simulink model "lab1simulink"  (R2021a)
settings: Solver=VariableStepAuto  StartTime=0.0  StopTime=80  RelTol=1e-3
undefined symbols (not defined in the file): c, d, g, J, L, m
libraries: fuzblock x2, simulink_extras x2
settings Model: Creator=ejbejaranos  LastModifiedBy=ejbejaranos

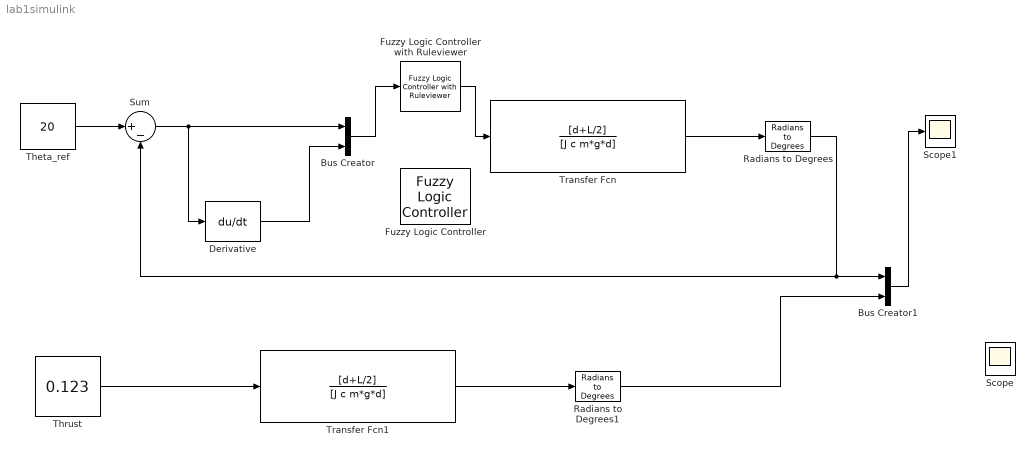
== system lab1simulink ==
  Bus Creator : BusCreator  Inputs=2
  Bus Creator1 : BusCreator  Inputs=2
  Derivative : Derivative
  Fuzzy Logic Controller : fuzblock/Fuzzy Logic  Controller  FIS=Fuzzy  OutputSampleNumber=101  DataType=double  FuzzifiedInputs=off  RuleFiringStrengths=off  RuleOutputs=off  AggregatedOutputs=off  SimulateUsing=Interpreted execution  OutOfRangeInputValueMessage=warning  NoRuleFiredMessage=warning  EmptyOutputFuzzySetMessage=warning
  Fuzzy Logic Controller with Ruleviewer : fuzblock/Fuzzy Logic  Controller  with Ruleviewer  fismatrix=Fuzzy  Ts=2
  Radians to Degrees : simulink_extras/Transformations/Radians to Degrees
  Radians to Degrees1 : simulink_extras/Transformations/Radians to Degrees
  Scope : Scope  NumInputPorts=2
  Scope1 : Scope
  Sum : Sum  Inputs=|+-
  Theta_ref : Constant  Value=20
  Thrust : Constant  Value=0.123
  Transfer Fcn : TransferFcn  Numerator=[d+L/2]  Denominator=[J c m*g*d]
  Transfer Fcn1 : TransferFcn  Numerator=[d+L/2]  Denominator=[J c m*g*d]
  wires:
  Theta_ref/1 -> Sum/1
  Bus Creator/1 -> Fuzzy Logic Controller with Ruleviewer/1
  Sum/1 -> Bus Creator/1, Derivative/1
  Derivative/1 -> Bus Creator/2
  Transfer Fcn/1 -> Radians to Degrees/1
  Radians to Degrees/1 -> Bus Creator1/1, Sum/2
  Thrust/1 -> Transfer Fcn1/1
  Transfer Fcn1/1 -> Radians to Degrees1/1
  Bus Creator1/1 -> Scope1/1
  Radians to Degrees1/1 -> Bus Creator1/2
  Fuzzy Logic Controller with Ruleviewer/1 -> Transfer Fcn/1
